simulink model "building_PHPP_v1"  (R2018b)
settings: Solver=ode23s  StartTime=-building.preruntime+8760*3600  StopTime=building.runtime+8760*3600  EnableMultiTasking=on
StartFcn:
  | tic
StopFcn:
  | toc
values from neighbouring files (symbols this model uses):
  A = 7*10*2    (= 140)    [theta_ground_v1.m]    (also in xlswrite1.m = num2cell(data))
  B = A/(0.5 * P)    (= 8.23529411765)    [theta_ground_v1.m]
  building = obj    [BUILDING.m]    (also in create_building_automatic.m = building.save(); ini_building_automatic.m = building.add_variant_hvac(building.variant_hvac, hvac); load_building_automatic.m = building.save())
  C = zeros(1,length(d)+1)    [CONSTRUCTION.m]    (also in DOOR.m = [0 0 0]; WALL.m = [0 0 0]; WINDOW.m = [0 0 0])
  cp = str2num(value)    [CONSTRUCTION.m]
  p = [timevec_weather weather(:,12)]    [BOUNDARY.m]    (also in WEATHER.m = 0; init_carnotUIBK.m = cell2mat(carnotUIBKpaths(i,2)))
  rho = str2num(value)    [CONSTRUCTION.m]    (also in theta_ground_v1.m = 2000)
undefined symbols (not defined in the file or in its folder): Dd, Dreifach, get_building, Qdot_C, Qdot_C_energy, Qdot_H, Qdot_H_energy, Qdot_I_electricity, Qdot_I_electricity_energy, Qdot_I_light, Qdot_I_light_energy, Qdot_I_person, Qdot_I_person_energy, Qdot_S, Qdot_S_energy, Qdot_T_ground, Qdot_T_ground_energy, Qdot_T_neighbour, Qdot_T_neighbour_energy, Qdot_T_opaque, Qdot_T_opaque_energy, Qdot_T_window, Qdot_T_window_energy, Qdot_V_infiltration, Qdot_V_infiltration_energy, Qdot_V_mech, Qdot_V_mech_energy, Qdot_V_window, Qdot_V_window_energy, Tc, Tr, Ts, Wärmeschutzglas, x_CO2, x_H2O, x_VOC
libraries: carnotUIBK x1874, carnot x5, simulink x3
(part 4 of 34)

== system building_PHPP_v1/BUILDING/INTERSECTION_2_7 ==
  AIB1 : Inport
  AIB2 : Inport  Port=2
  BDB1 : Inport  Port=3
  BDB2 : Inport  Port=4
  control : Inport  Port=5
  Add : Sum  Inputs=++++++
  Add1 : Sum  Inputs=++++++
  Bus Selector : BusSelector  OutputSignals=Qdot_S
  Bus Selector1 : BusSelector  OutputSignals=Qdot_S
  airexchange_1 : Subsystem  Variant=on  mask{zone=i.matrix_wd, window=1}
      mask prompts: window "wall"
      mask init: same as building_PHPP_v1/BUILDING/INTERSECTION_1_10/airexchange_1
      mask Display:
      | fprintf('AIR EXCHANGE\n')
      | %fprintf('\n%s', const.name)
  airexchange_2 : Subsystem  Variant=on  mask{zone=i.matrix_wd, window=2}
      mask prompts: window "wall"
      mask init: same as building_PHPP_v1/BUILDING/INTERSECTION_1_10/airexchange_1
      mask Display:
      | fprintf('AIR EXCHANGE\n')
      | %fprintf('\n%s', const.name)
  airexchange_3 : Subsystem  Variant=on  mask{zone=i.matrix_wd, window=3}
      mask prompts: window "wall"
      mask init: same as building_PHPP_v1/BUILDING/INTERSECTION_1_10/airexchange_1
      mask Display:
      | fprintf('AIR EXCHANGE\n')
      | %fprintf('\n%s', const.name)
  wall_1 : Subsystem  Variant=on  mask{zone=i.matrix_wd, construction=b.construction, wall=1}
      mask init: same as building_PHPP_v1/BUILDING/INTERSECTION_1_10/wall_1
      mask Display:
      | fprintf('CONSTRUCTION:\n')
      | fprintf('\n%s', const.name)
  wall_2 : Subsystem  Variant=on  mask{zone=i.matrix_wd, construction=b.construction, wall=2}
      mask init: same as building_PHPP_v1/BUILDING/INTERSECTION_1_10/wall_1
      mask Display:
      | fprintf('CONSTRUCTION:\n')
      | fprintf('\n%s', const.name)
  wall_3 : Subsystem  Variant=on  mask{zone=i.matrix_wd, construction=b.construction, wall=3}
      mask init: same as building_PHPP_v1/BUILDING/INTERSECTION_1_10/wall_1
      mask Display:
      | fprintf('CONSTRUCTION:\n')
      | fprintf('\n%s', const.name)
  S1 : Outport
  S2 : Outport  Port=2
  wires:
  Add/1 -> S1/1
  Add1/1 -> S2/1
  BDB1/1 -> Bus Selector/1
  Bus Selector/1 -> wall_1/3(Qdot_sol1), wall_2/3(Qdot_sol1), wall_3/3(Qdot_sol1)  "<Qdot_S>"
  BDB2/1 -> Bus Selector1/1
  Bus Selector1/1 -> wall_1/4(Qdot_sol2), wall_2/4(Qdot_sol2), wall_3/4(Qdot_sol2)  "<Qdot_S>"
  control/1 -> airexchange_3/3(control), airexchange_2/3(control), airexchange_1/3(control)
  AIB2/1 -> wall_2/2(AIB2), wall_3/2(AIB2), airexchange_3/2(AIB2), airexchange_2/2(AIB2), airexchange_1/2(AIB2), wall_1/2(AIB2)
  AIB1/1 -> wall_2/1(AIB1), wall_3/1(AIB1), airexchange_3/1(AIB1), airexchange_2/1(AIB1), airexchange_1/1(AIB1), wall_1/1(AIB1)
  wall_1/1("[S1]") -> Add/1
  wall_2/1("[S1]") -> Add/2
  wall_3/1("[S1]") -> Add/3
  airexchange_1/1("[S1]") -> Add/4
  airexchange_2/1("[S1]") -> Add/5
  airexchange_3/1("[S1]") -> Add/6
  wall_1/2("[S2]") -> Add1/1
  wall_2/2("[S2]") -> Add1/2
  airexchange_3/2("[S2]") -> Add1/6
  airexchange_2/2("[S2]") -> Add1/5
  airexchange_1/2("[S2]") -> Add1/4
  wall_3/2("[S2]") -> Add1/3

== system building_PHPP_v1/BUILDING/INTERSECTION_2_8 ==
  AIB1 : Inport
  AIB2 : Inport  Port=2
  BDB1 : Inport  Port=3
  BDB2 : Inport  Port=4
  control : Inport  Port=5
  Add : Sum  Inputs=++++++
  Add1 : Sum  Inputs=++++++
  Bus Selector : BusSelector  OutputSignals=Qdot_S
  Bus Selector1 : BusSelector  OutputSignals=Qdot_S
  airexchange_1 : Subsystem  Variant=on  mask{zone=i.matrix_wd, window=1}
      mask prompts: window "wall"
      mask init: same as building_PHPP_v1/BUILDING/INTERSECTION_1_10/airexchange_1
      mask Display:
      | fprintf('AIR EXCHANGE\n')
      | %fprintf('\n%s', const.name)
  airexchange_2 : Subsystem  Variant=on  mask{zone=i.matrix_wd, window=2}
      mask prompts: window "wall"
      mask init: same as building_PHPP_v1/BUILDING/INTERSECTION_1_10/airexchange_1
      mask Display:
      | fprintf('AIR EXCHANGE\n')
      | %fprintf('\n%s', const.name)
  airexchange_3 : Subsystem  Variant=on  mask{zone=i.matrix_wd, window=3}
      mask prompts: window "wall"
      mask init: same as building_PHPP_v1/BUILDING/INTERSECTION_1_10/airexchange_1
      mask Display:
      | fprintf('AIR EXCHANGE\n')
      | %fprintf('\n%s', const.name)
  wall_1 : Subsystem  Variant=on  mask{zone=i.matrix_wd, construction=b.construction, wall=1}
      mask init: same as building_PHPP_v1/BUILDING/INTERSECTION_1_10/wall_1
      mask Display:
      | fprintf('CONSTRUCTION:\n')
      | fprintf('\n%s', const.name)
  wall_2 : Subsystem  Variant=on  mask{zone=i.matrix_wd, construction=b.construction, wall=2}
      mask init: same as building_PHPP_v1/BUILDING/INTERSECTION_1_10/wall_1
      mask Display:
      | fprintf('CONSTRUCTION:\n')
      | fprintf('\n%s', const.name)
  wall_3 : Subsystem  Variant=on  mask{zone=i.matrix_wd, construction=b.construction, wall=3}
      mask init: same as building_PHPP_v1/BUILDING/INTERSECTION_1_10/wall_1
      mask Display:
      | fprintf('CONSTRUCTION:\n')
      | fprintf('\n%s', const.name)
  S1 : Outport
  S2 : Outport  Port=2
  wires:
  Add/1 -> S1/1
  Add1/1 -> S2/1
  BDB1/1 -> Bus Selector/1
  Bus Selector/1 -> wall_1/3(Qdot_sol1), wall_2/3(Qdot_sol1), wall_3/3(Qdot_sol1)  "<Qdot_S>"
  BDB2/1 -> Bus Selector1/1
  Bus Selector1/1 -> wall_1/4(Qdot_sol2), wall_2/4(Qdot_sol2), wall_3/4(Qdot_sol2)  "<Qdot_S>"
  control/1 -> airexchange_3/3(control), airexchange_2/3(control), airexchange_1/3(control)
  AIB2/1 -> wall_2/2(AIB2), wall_3/2(AIB2), airexchange_3/2(AIB2), airexchange_2/2(AIB2), airexchange_1/2(AIB2), wall_1/2(AIB2)
  AIB1/1 -> wall_2/1(AIB1), wall_3/1(AIB1), airexchange_3/1(AIB1), airexchange_2/1(AIB1), airexchange_1/1(AIB1), wall_1/1(AIB1)
  wall_1/1("[S1]") -> Add/1
  wall_2/1("[S1]") -> Add/2
  wall_3/1("[S1]") -> Add/3
  airexchange_1/1("[S1]") -> Add/4
  airexchange_2/1("[S1]") -> Add/5
  airexchange_3/1("[S1]") -> Add/6
  wall_1/2("[S2]") -> Add1/1
  wall_2/2("[S2]") -> Add1/2
  airexchange_3/2("[S2]") -> Add1/6
  airexchange_2/2("[S2]") -> Add1/5
  airexchange_1/2("[S2]") -> Add1/4
  wall_3/2("[S2]") -> Add1/3

== system building_PHPP_v1/BUILDING/INTERSECTION_2_9 ==
  AIB1 : Inport
  AIB2 : Inport  Port=2
  BDB1 : Inport  Port=3
  BDB2 : Inport  Port=4
  control : Inport  Port=5
  Add : Sum  Inputs=++++++
  Add1 : Sum  Inputs=++++++
  Bus Selector : BusSelector  OutputSignals=Qdot_S
  Bus Selector1 : BusSelector  OutputSignals=Qdot_S
  airexchange_1 : Subsystem  Variant=on  mask{zone=i.matrix_wd, window=1}
      mask prompts: window "wall"
      mask init: same as building_PHPP_v1/BUILDING/INTERSECTION_1_10/airexchange_1
      mask Display:
      | fprintf('AIR EXCHANGE\n')
      | %fprintf('\n%s', const.name)
  airexchange_2 : Subsystem  Variant=on  mask{zone=i.matrix_wd, window=2}
      mask prompts: window "wall"
      mask init: same as building_PHPP_v1/BUILDING/INTERSECTION_1_10/airexchange_1
      mask Display:
      | fprintf('AIR EXCHANGE\n')
      | %fprintf('\n%s', const.name)
  airexchange_3 : Subsystem  Variant=on  mask{zone=i.matrix_wd, window=3}
      mask prompts: window "wall"
      mask init: same as building_PHPP_v1/BUILDING/INTERSECTION_1_10/airexchange_1
      mask Display:
      | fprintf('AIR EXCHANGE\n')
      | %fprintf('\n%s', const.name)
  wall_1 : Subsystem  Variant=on  mask{zone=i.matrix_wd, construction=b.construction, wall=1}
      mask init: same as building_PHPP_v1/BUILDING/INTERSECTION_1_10/wall_1
      mask Display:
      | fprintf('CONSTRUCTION:\n')
      | fprintf('\n%s', const.name)
  wall_2 : Subsystem  Variant=on  mask{zone=i.matrix_wd, construction=b.construction, wall=2}
      mask init: same as building_PHPP_v1/BUILDING/INTERSECTION_1_10/wall_1
      mask Display:
      | fprintf('CONSTRUCTION:\n')
      | fprintf('\n%s', const.name)
  wall_3 : Subsystem  Variant=on  mask{zone=i.matrix_wd, construction=b.construction, wall=3}
      mask init: same as building_PHPP_v1/BUILDING/INTERSECTION_1_10/wall_1
      mask Display:
      | fprintf('CONSTRUCTION:\n')
      | fprintf('\n%s', const.name)
  S1 : Outport
  S2 : Outport  Port=2
  wires:
  Add/1 -> S1/1
  Add1/1 -> S2/1
  BDB1/1 -> Bus Selector/1
  Bus Selector/1 -> wall_1/3(Qdot_sol1), wall_2/3(Qdot_sol1), wall_3/3(Qdot_sol1)  "<Qdot_S>"
  BDB2/1 -> Bus Selector1/1
  Bus Selector1/1 -> wall_1/4(Qdot_sol2), wall_2/4(Qdot_sol2), wall_3/4(Qdot_sol2)  "<Qdot_S>"
  control/1 -> airexchange_3/3(control), airexchange_2/3(control), airexchange_1/3(control)
  AIB2/1 -> wall_2/2(AIB2), wall_3/2(AIB2), airexchange_3/2(AIB2), airexchange_2/2(AIB2), airexchange_1/2(AIB2), wall_1/2(AIB2)
  AIB1/1 -> wall_2/1(AIB1), wall_3/1(AIB1), airexchange_3/1(AIB1), airexchange_2/1(AIB1), airexchange_1/1(AIB1), wall_1/1(AIB1)
  wall_1/1("[S1]") -> Add/1
  wall_2/1("[S1]") -> Add/2
  wall_3/1("[S1]") -> Add/3
  airexchange_1/1("[S1]") -> Add/4
  airexchange_2/1("[S1]") -> Add/5
  airexchange_3/1("[S1]") -> Add/6
  wall_1/2("[S2]") -> Add1/1
  wall_2/2("[S2]") -> Add1/2
  airexchange_3/2("[S2]") -> Add1/6
  airexchange_2/2("[S2]") -> Add1/5
  airexchange_1/2("[S2]") -> Add1/4
  wall_3/2("[S2]") -> Add1/3

== system building_PHPP_v1/BUILDING/INTERSECTION_3_10 ==
  AIB1 : Inport
  AIB2 : Inport  Port=2
  BDB1 : Inport  Port=3
  BDB2 : Inport  Port=4
  control : Inport  Port=5
  Add : Sum  Inputs=++++++
  Add1 : Sum  Inputs=++++++
  Bus Selector : BusSelector  OutputSignals=Qdot_S
  Bus Selector1 : BusSelector  OutputSignals=Qdot_S
  airexchange_1 : Subsystem  Variant=on  mask{zone=i.matrix_wd, window=1}
      mask prompts: window "wall"
      mask init: same as building_PHPP_v1/BUILDING/INTERSECTION_1_10/airexchange_1
      mask Display:
      | fprintf('AIR EXCHANGE\n')
      | %fprintf('\n%s', const.name)
  airexchange_2 : Subsystem  Variant=on  mask{zone=i.matrix_wd, window=2}
      mask prompts: window "wall"
      mask init: same as building_PHPP_v1/BUILDING/INTERSECTION_1_10/airexchange_1
      mask Display:
      | fprintf('AIR EXCHANGE\n')
      | %fprintf('\n%s', const.name)
  airexchange_3 : Subsystem  Variant=on  mask{zone=i.matrix_wd, window=3}
      mask prompts: window "wall"
      mask init: same as building_PHPP_v1/BUILDING/INTERSECTION_1_10/airexchange_1
      mask Display:
      | fprintf('AIR EXCHANGE\n')
      | %fprintf('\n%s', const.name)
  wall_1 : Subsystem  Variant=on  mask{zone=i.matrix_wd, construction=b.construction, wall=1}
      mask init: same as building_PHPP_v1/BUILDING/INTERSECTION_1_10/wall_1
      mask Display:
      | fprintf('CONSTRUCTION:\n')
      | fprintf('\n%s', const.name)
  wall_2 : Subsystem  Variant=on  mask{zone=i.matrix_wd, construction=b.construction, wall=2}
      mask init: same as building_PHPP_v1/BUILDING/INTERSECTION_1_10/wall_1
      mask Display:
      | fprintf('CONSTRUCTION:\n')
      | fprintf('\n%s', const.name)
  wall_3 : Subsystem  Variant=on  mask{zone=i.matrix_wd, construction=b.construction, wall=3}
      mask init: same as building_PHPP_v1/BUILDING/INTERSECTION_1_10/wall_1
      mask Display:
      | fprintf('CONSTRUCTION:\n')
      | fprintf('\n%s', const.name)
  S1 : Outport
  S2 : Outport  Port=2
  wires:
  Add/1 -> S1/1
  Add1/1 -> S2/1
  BDB1/1 -> Bus Selector/1
  Bus Selector/1 -> wall_1/3(Qdot_sol1), wall_2/3(Qdot_sol1), wall_3/3(Qdot_sol1)  "<Qdot_S>"
  BDB2/1 -> Bus Selector1/1
  Bus Selector1/1 -> wall_1/4(Qdot_sol2), wall_2/4(Qdot_sol2), wall_3/4(Qdot_sol2)  "<Qdot_S>"
  control/1 -> airexchange_3/3(control), airexchange_2/3(control), airexchange_1/3(control)
  AIB2/1 -> wall_2/2(AIB2), wall_3/2(AIB2), airexchange_3/2(AIB2), airexchange_2/2(AIB2), airexchange_1/2(AIB2), wall_1/2(AIB2)
  AIB1/1 -> wall_2/1(AIB1), wall_3/1(AIB1), airexchange_3/1(AIB1), airexchange_2/1(AIB1), airexchange_1/1(AIB1), wall_1/1(AIB1)
  wall_1/1("[S1]") -> Add/1
  wall_2/1("[S1]") -> Add/2
  wall_3/1("[S1]") -> Add/3
  airexchange_1/1("[S1]") -> Add/4
  airexchange_2/1("[S1]") -> Add/5
  airexchange_3/1("[S1]") -> Add/6
  wall_1/2("[S2]") -> Add1/1
  wall_2/2("[S2]") -> Add1/2
  airexchange_3/2("[S2]") -> Add1/6
  airexchange_2/2("[S2]") -> Add1/5
  airexchange_1/2("[S2]") -> Add1/4
  wall_3/2("[S2]") -> Add1/3

== system building_PHPP_v1/BUILDING/INTERSECTION_3_4 ==
  AIB1 : Inport
  AIB2 : Inport  Port=2
  BDB1 : Inport  Port=3
  BDB2 : Inport  Port=4
  control : Inport  Port=5
  Add : Sum  Inputs=++++++
  Add1 : Sum  Inputs=++++++
  Bus Selector : BusSelector  OutputSignals=Qdot_S
  Bus Selector1 : BusSelector  OutputSignals=Qdot_S
  airexchange_1 : Subsystem  Variant=on  mask{zone=i.matrix_wd, window=1}
      mask prompts: window "wall"
      mask init: same as building_PHPP_v1/BUILDING/INTERSECTION_1_10/airexchange_1
      mask Display:
      | fprintf('AIR EXCHANGE\n')
      | %fprintf('\n%s', const.name)
  airexchange_2 : Subsystem  Variant=on  mask{zone=i.matrix_wd, window=2}
      mask prompts: window "wall"
      mask init: same as building_PHPP_v1/BUILDING/INTERSECTION_1_10/airexchange_1
      mask Display:
      | fprintf('AIR EXCHANGE\n')
      | %fprintf('\n%s', const.name)
  airexchange_3 : Subsystem  Variant=on  mask{zone=i.matrix_wd, window=3}
      mask prompts: window "wall"
      mask init: same as building_PHPP_v1/BUILDING/INTERSECTION_1_10/airexchange_1
      mask Display:
      | fprintf('AIR EXCHANGE\n')
      | %fprintf('\n%s', const.name)
  wall_1 : Subsystem  Variant=on  mask{zone=i.matrix_wd, construction=b.construction, wall=1}
      mask init: same as building_PHPP_v1/BUILDING/INTERSECTION_1_10/wall_1
      mask Display:
      | fprintf('CONSTRUCTION:\n')
      | fprintf('\n%s', const.name)
  wall_2 : Subsystem  Variant=on  mask{zone=i.matrix_wd, construction=b.construction, wall=2}
      mask init: same as building_PHPP_v1/BUILDING/INTERSECTION_1_10/wall_1
      mask Display:
      | fprintf('CONSTRUCTION:\n')
      | fprintf('\n%s', const.name)
  wall_3 : Subsystem  Variant=on  mask{zone=i.matrix_wd, construction=b.construction, wall=3}
      mask init: same as building_PHPP_v1/BUILDING/INTERSECTION_1_10/wall_1
      mask Display:
      | fprintf('CONSTRUCTION:\n')
      | fprintf('\n%s', const.name)
  S1 : Outport
  S2 : Outport  Port=2
  wires:
  Add/1 -> S1/1
  Add1/1 -> S2/1
  BDB1/1 -> Bus Selector/1
  Bus Selector/1 -> wall_1/3(Qdot_sol1), wall_2/3(Qdot_sol1), wall_3/3(Qdot_sol1)  "<Qdot_S>"
  BDB2/1 -> Bus Selector1/1
  Bus Selector1/1 -> wall_1/4(Qdot_sol2), wall_2/4(Qdot_sol2), wall_3/4(Qdot_sol2)  "<Qdot_S>"
  control/1 -> airexchange_3/3(control), airexchange_2/3(control), airexchange_1/3(control)
  AIB2/1 -> wall_2/2(AIB2), wall_3/2(AIB2), airexchange_3/2(AIB2), airexchange_2/2(AIB2), airexchange_1/2(AIB2), wall_1/2(AIB2)
  AIB1/1 -> wall_2/1(AIB1), wall_3/1(AIB1), airexchange_3/1(AIB1), airexchange_2/1(AIB1), airexchange_1/1(AIB1), wall_1/1(AIB1)
  wall_1/1("[S1]") -> Add/1
  wall_2/1("[S1]") -> Add/2
  wall_3/1("[S1]") -> Add/3
  airexchange_1/1("[S1]") -> Add/4
  airexchange_2/1("[S1]") -> Add/5
  airexchange_3/1("[S1]") -> Add/6
  wall_1/2("[S2]") -> Add1/1
  wall_2/2("[S2]") -> Add1/2
  airexchange_3/2("[S2]") -> Add1/6
  airexchange_2/2("[S2]") -> Add1/5
  airexchange_1/2("[S2]") -> Add1/4
  wall_3/2("[S2]") -> Add1/3

== system building_PHPP_v1/BUILDING/INTERSECTION_3_5 ==
  AIB1 : Inport
  AIB2 : Inport  Port=2
  BDB1 : Inport  Port=3
  BDB2 : Inport  Port=4
  control : Inport  Port=5
  Add : Sum  Inputs=++++++
  Add1 : Sum  Inputs=++++++
  Bus Selector : BusSelector  OutputSignals=Qdot_S
  Bus Selector1 : BusSelector  OutputSignals=Qdot_S
  airexchange_1 : Subsystem  Variant=on  mask{zone=i.matrix_wd, window=1}
      mask prompts: window "wall"
      mask init: same as building_PHPP_v1/BUILDING/INTERSECTION_1_10/airexchange_1
      mask Display:
      | fprintf('AIR EXCHANGE\n')
      | %fprintf('\n%s', const.name)
  airexchange_2 : Subsystem  Variant=on  mask{zone=i.matrix_wd, window=2}
      mask prompts: window "wall"
      mask init: same as building_PHPP_v1/BUILDING/INTERSECTION_1_10/airexchange_1
      mask Display:
      | fprintf('AIR EXCHANGE\n')
      | %fprintf('\n%s', const.name)
  airexchange_3 : Subsystem  Variant=on  mask{zone=i.matrix_wd, window=3}
      mask prompts: window "wall"
      mask init: same as building_PHPP_v1/BUILDING/INTERSECTION_1_10/airexchange_1
      mask Display:
      | fprintf('AIR EXCHANGE\n')
      | %fprintf('\n%s', const.name)
  wall_1 : Subsystem  Variant=on  mask{zone=i.matrix_wd, construction=b.construction, wall=1}
      mask init: same as building_PHPP_v1/BUILDING/INTERSECTION_1_10/wall_1
      mask Display:
      | fprintf('CONSTRUCTION:\n')
      | fprintf('\n%s', const.name)
  wall_2 : Subsystem  Variant=on  mask{zone=i.matrix_wd, construction=b.construction, wall=2}
      mask init: same as building_PHPP_v1/BUILDING/INTERSECTION_1_10/wall_1
      mask Display:
      | fprintf('CONSTRUCTION:\n')
      | fprintf('\n%s', const.name)
  wall_3 : Subsystem  Variant=on  mask{zone=i.matrix_wd, construction=b.construction, wall=3}
      mask init: same as building_PHPP_v1/BUILDING/INTERSECTION_1_10/wall_1
      mask Display:
      | fprintf('CONSTRUCTION:\n')
      | fprintf('\n%s', const.name)
  S1 : Outport
  S2 : Outport  Port=2
  wires:
  Add/1 -> S1/1
  Add1/1 -> S2/1
  BDB1/1 -> Bus Selector/1
  Bus Selector/1 -> wall_1/3(Qdot_sol1), wall_2/3(Qdot_sol1), wall_3/3(Qdot_sol1)  "<Qdot_S>"
  BDB2/1 -> Bus Selector1/1
  Bus Selector1/1 -> wall_1/4(Qdot_sol2), wall_2/4(Qdot_sol2), wall_3/4(Qdot_sol2)  "<Qdot_S>"
  control/1 -> airexchange_3/3(control), airexchange_2/3(control), airexchange_1/3(control)
  AIB2/1 -> wall_2/2(AIB2), wall_3/2(AIB2), airexchange_3/2(AIB2), airexchange_2/2(AIB2), airexchange_1/2(AIB2), wall_1/2(AIB2)
  AIB1/1 -> wall_2/1(AIB1), wall_3/1(AIB1), airexchange_3/1(AIB1), airexchange_2/1(AIB1), airexchange_1/1(AIB1), wall_1/1(AIB1)
  wall_1/1("[S1]") -> Add/1
  wall_2/1("[S1]") -> Add/2
  wall_3/1("[S1]") -> Add/3
  airexchange_1/1("[S1]") -> Add/4
  airexchange_2/1("[S1]") -> Add/5
  airexchange_3/1("[S1]") -> Add/6
  wall_1/2("[S2]") -> Add1/1
  wall_2/2("[S2]") -> Add1/2
  airexchange_3/2("[S2]") -> Add1/6
  airexchange_2/2("[S2]") -> Add1/5
  airexchange_1/2("[S2]") -> Add1/4
  wall_3/2("[S2]") -> Add1/3

== system building_PHPP_v1/BUILDING/INTERSECTION_3_6 ==
  AIB1 : Inport
  AIB2 : Inport  Port=2
  BDB1 : Inport  Port=3
  BDB2 : Inport  Port=4
  control : Inport  Port=5
  Add : Sum  Inputs=++++++
  Add1 : Sum  Inputs=++++++
  Bus Selector : BusSelector  OutputSignals=Qdot_S
  Bus Selector1 : BusSelector  OutputSignals=Qdot_S
  airexchange_1 : Subsystem  Variant=on  mask{zone=i.matrix_wd, window=1}
      mask prompts: window "wall"
      mask init: same as building_PHPP_v1/BUILDING/INTERSECTION_1_10/airexchange_1
      mask Display:
      | fprintf('AIR EXCHANGE\n')
      | %fprintf('\n%s', const.name)
  airexchange_2 : Subsystem  Variant=on  mask{zone=i.matrix_wd, window=2}
      mask prompts: window "wall"
      mask init: same as building_PHPP_v1/BUILDING/INTERSECTION_1_10/airexchange_1
      mask Display:
      | fprintf('AIR EXCHANGE\n')
      | %fprintf('\n%s', const.name)
  airexchange_3 : Subsystem  Variant=on  mask{zone=i.matrix_wd, window=3}
      mask prompts: window "wall"
      mask init: same as building_PHPP_v1/BUILDING/INTERSECTION_1_10/airexchange_1
      mask Display:
      | fprintf('AIR EXCHANGE\n')
      | %fprintf('\n%s', const.name)
  wall_1 : Subsystem  Variant=on  mask{zone=i.matrix_wd, construction=b.construction, wall=1}
      mask init: same as building_PHPP_v1/BUILDING/INTERSECTION_1_10/wall_1
      mask Display:
      | fprintf('CONSTRUCTION:\n')
      | fprintf('\n%s', const.name)
  wall_2 : Subsystem  Variant=on  mask{zone=i.matrix_wd, construction=b.construction, wall=2}
      mask init: same as building_PHPP_v1/BUILDING/INTERSECTION_1_10/wall_1
      mask Display:
      | fprintf('CONSTRUCTION:\n')
      | fprintf('\n%s', const.name)
  wall_3 : Subsystem  Variant=on  mask{zone=i.matrix_wd, construction=b.construction, wall=3}
      mask init: same as building_PHPP_v1/BUILDING/INTERSECTION_1_10/wall_1
      mask Display:
      | fprintf('CONSTRUCTION:\n')
      | fprintf('\n%s', const.name)
  S1 : Outport
  S2 : Outport  Port=2
  wires:
  Add/1 -> S1/1
  Add1/1 -> S2/1
  BDB1/1 -> Bus Selector/1
  Bus Selector/1 -> wall_1/3(Qdot_sol1), wall_2/3(Qdot_sol1), wall_3/3(Qdot_sol1)  "<Qdot_S>"
  BDB2/1 -> Bus Selector1/1
  Bus Selector1/1 -> wall_1/4(Qdot_sol2), wall_2/4(Qdot_sol2), wall_3/4(Qdot_sol2)  "<Qdot_S>"
  control/1 -> airexchange_3/3(control), airexchange_2/3(control), airexchange_1/3(control)
  AIB2/1 -> wall_2/2(AIB2), wall_3/2(AIB2), airexchange_3/2(AIB2), airexchange_2/2(AIB2), airexchange_1/2(AIB2), wall_1/2(AIB2)
  AIB1/1 -> wall_2/1(AIB1), wall_3/1(AIB1), airexchange_3/1(AIB1), airexchange_2/1(AIB1), airexchange_1/1(AIB1), wall_1/1(AIB1)
  wall_1/1("[S1]") -> Add/1
  wall_2/1("[S1]") -> Add/2
  wall_3/1("[S1]") -> Add/3
  airexchange_1/1("[S1]") -> Add/4
  airexchange_2/1("[S1]") -> Add/5
  airexchange_3/1("[S1]") -> Add/6
  wall_1/2("[S2]") -> Add1/1
  wall_2/2("[S2]") -> Add1/2
  airexchange_3/2("[S2]") -> Add1/6
  airexchange_2/2("[S2]") -> Add1/5
  airexchange_1/2("[S2]") -> Add1/4
  wall_3/2("[S2]") -> Add1/3

== system building_PHPP_v1/BUILDING/INTERSECTION_3_7 ==
  AIB1 : Inport
  AIB2 : Inport  Port=2
  BDB1 : Inport  Port=3
  BDB2 : Inport  Port=4
  control : Inport  Port=5
  Add : Sum  Inputs=++++++
  Add1 : Sum  Inputs=++++++
  Bus Selector : BusSelector  OutputSignals=Qdot_S
  Bus Selector1 : BusSelector  OutputSignals=Qdot_S
  airexchange_1 : Subsystem  Variant=on  mask{zone=i.matrix_wd, window=1}
      mask prompts: window "wall"
      mask init: same as building_PHPP_v1/BUILDING/INTERSECTION_1_10/airexchange_1
      mask Display:
      | fprintf('AIR EXCHANGE\n')
      | %fprintf('\n%s', const.name)
  airexchange_2 : Subsystem  Variant=on  mask{zone=i.matrix_wd, window=2}
      mask prompts: window "wall"
      mask init: same as building_PHPP_v1/BUILDING/INTERSECTION_1_10/airexchange_1
      mask Display:
      | fprintf('AIR EXCHANGE\n')
      | %fprintf('\n%s', const.name)
  airexchange_3 : Subsystem  Variant=on  mask{zone=i.matrix_wd, window=3}
      mask prompts: window "wall"
      mask init: same as building_PHPP_v1/BUILDING/INTERSECTION_1_10/airexchange_1
      mask Display:
      | fprintf('AIR EXCHANGE\n')
      | %fprintf('\n%s', const.name)
  wall_1 : Subsystem  Variant=on  mask{zone=i.matrix_wd, construction=b.construction, wall=1}
      mask init: same as building_PHPP_v1/BUILDING/INTERSECTION_1_10/wall_1
      mask Display:
      | fprintf('CONSTRUCTION:\n')
      | fprintf('\n%s', const.name)
  wall_2 : Subsystem  Variant=on  mask{zone=i.matrix_wd, construction=b.construction, wall=2}
      mask init: same as building_PHPP_v1/BUILDING/INTERSECTION_1_10/wall_1
      mask Display:
      | fprintf('CONSTRUCTION:\n')
      | fprintf('\n%s', const.name)
  wall_3 : Subsystem  Variant=on  mask{zone=i.matrix_wd, construction=b.construction, wall=3}
      mask init: same as building_PHPP_v1/BUILDING/INTERSECTION_1_10/wall_1
      mask Display:
      | fprintf('CONSTRUCTION:\n')
      | fprintf('\n%s', const.name)
  S1 : Outport
  S2 : Outport  Port=2
  wires:
  Add/1 -> S1/1
  Add1/1 -> S2/1
  BDB1/1 -> Bus Selector/1
  Bus Selector/1 -> wall_1/3(Qdot_sol1), wall_2/3(Qdot_sol1), wall_3/3(Qdot_sol1)  "<Qdot_S>"
  BDB2/1 -> Bus Selector1/1
  Bus Selector1/1 -> wall_1/4(Qdot_sol2), wall_2/4(Qdot_sol2), wall_3/4(Qdot_sol2)  "<Qdot_S>"
  control/1 -> airexchange_3/3(control), airexchange_2/3(control), airexchange_1/3(control)
  AIB2/1 -> wall_2/2(AIB2), wall_3/2(AIB2), airexchange_3/2(AIB2), airexchange_2/2(AIB2), airexchange_1/2(AIB2), wall_1/2(AIB2)
  AIB1/1 -> wall_2/1(AIB1), wall_3/1(AIB1), airexchange_3/1(AIB1), airexchange_2/1(AIB1), airexchange_1/1(AIB1), wall_1/1(AIB1)
  wall_1/1("[S1]") -> Add/1
  wall_2/1("[S1]") -> Add/2
  wall_3/1("[S1]") -> Add/3
  airexchange_1/1("[S1]") -> Add/4
  airexchange_2/1("[S1]") -> Add/5
  airexchange_3/1("[S1]") -> Add/6
  wall_1/2("[S2]") -> Add1/1
  wall_2/2("[S2]") -> Add1/2
  airexchange_3/2("[S2]") -> Add1/6
  airexchange_2/2("[S2]") -> Add1/5
  airexchange_1/2("[S2]") -> Add1/4
  wall_3/2("[S2]") -> Add1/3
